simulink model "DCV_test"  (R2025b)
settings: Solver=VariableStepAuto  StartTime=0.0  StopTime=10.0  RelTol=1e-3
model workspace (MATLAB code in the model file):
  | clear;
  | %% Hydraulics
  | 
  | %Liquid
  | rho = 875;
  | beta = 1000; %MPa
  | 
  | %Pump
  | pP = 10e6; %100 bar i pascal, velger den sjøl med å skru
  | 
  | %-------------------DCV-----------------------
  | dp0 = 20e5; %Nominal pressure drop, Pa
  | Q0 = 18/6e4; %Nominal flow, m^3/s
  | Cd = 0.55; %Discharge coefficient
  | AdMax_SI = Q0/(Cd*(2/rho*dp0)^0.5); %Discharge area m^2
  | AdMax = AdMax_SI*1e6;
  | 
  | %% DCV Orifice Area Vectors
  | 
  | % Deadband control signal thresholds
  | u_dead_up    = 0.236;
  | u_dead_down  = 0.206;
  | 
  | % Spool position at deadband
  | spool_dead_up   = 1.1182 * u_dead_up   - 0.0325;
  | spool_dead_down = 1.1075 * u_dead_down - 0.0416;
  | 
  | % Polynomial: spool position as function of Kv [L/min/sqrt(bar)]
  | % Valid from u = 0.25 to max stroke
  | p_spool_of_Kv_up   = [0.0018653, -0.033672,  0.22033, -0.65618,  0.83411, -0.047269, 0.26252];
  | p_spool_of_Kv_down = [0.00098272, -0.017507,  0.11599, -0.34851,  0.41222,  0.17643,  0.2076];
  | 
  | % Linear model slopes (from TwinCAT): spool_pos = spool_dead + slope * Kv
  | slope_Kv_up   = 0.270407;
  | slope_Kv_down = 0.230397;
  | 
  | % Evaluate polynomial over valid Kv range
  | Kv_range   = linspace(0.09, 4, 10000);
  | spool_up   = polyval(p_spool_of_Kv_up,   Kv_range);
  | spool_down = polyval(p_spool_of_Kv_down, Kv_range);
  | 
  | % Breakpoints: u = 0.25 to 0.50 in steps of 0.05, then max
  | %u_breakpoints = 0.25:0.05:1.0; tester flere punkter
  | u_breakpoints = [0.25, 0.30:0.025:1.0];
  | 
  | % Corresponding spool positions
  | spool_bp_up   = 1.1182 * u_breakpoints - 0.0325;
  | spool_bp_down = 1.1075 * u_breakpoints - 0.0416;
  | 
  | % Find Kv at each breakpoint using nearest-index lookup
  | Kv_bp_up   = zeros(1, length(u_breakpoints));
  | Kv_bp_down = zeros(1, length(u_breakpoints));
  | for i = 1:length(u_breakpoints)
  |     if u_breakpoints(i) <= 0.25
  |         % Use linear model for transition point
  |         Kv_bp_up(i)   = (spool_bp_up(i)   - spool_dead_up)   / slope_Kv_up;
  |         Kv_bp_down(i) = (spool_bp_down(i) - spool_dead_down) / slope_Kv_down;
  |     else
  |         % Use polynomial inversion via nearest-index lookup
  |         [~, idx_up]   = min(abs(spool_up   - spool_bp_up(i)));
  |         [~, idx_down] = min(abs(spool_down - spool_bp_down(i)));
  |         Kv_bp_up(i)   = Kv_range(idx_up);
  |         Kv_bp_down(i) = Kv_range(idx_down);
  |     end
  | end
  | 
  | % Kv at max spool
  | [~, idx_max_up]   = max(spool_up);
  | [~, idx_max_down] = max(spool_down);
  | Kv_max_up   = Kv_range(idx_max_up);
  | Kv_max_down = Kv_range(idx_max_down);
  | 
  | % Unit conversion: L/min/sqrt(bar) -> m³/s/sqrt(Pa)
  | Kv_unit_conv = sqrt(1e-5) / 6e4;
  | 
  | % Convert all Kv breakpoints to area [m²]
  | A_bp_up   = (Kv_bp_up   * Kv_unit_conv) / (Cd * sqrt(2/rho));
  | A_bp_down = (Kv_bp_down * Kv_unit_conv) / (Cd * sqrt(2/rho));
  | A_max_up  = (Kv_max_up  * Kv_unit_conv) / (Cd * sqrt(2/rho));
  | A_max_down= (Kv_max_down* Kv_unit_conv) / (Cd * sqrt(2/rho));
  | 
  | % Orifice area vectors [m²]: [leakage, crack-open, u=0.30...0.50, fully-open]
  | orifice_area_up   = [1e-9, A_bp_up,   A_max_up];
  | orifice_area_down = [1e-9, A_bp_down, A_max_down];
  | 
  | % Control member position vectors (must match area vectors one-to-one)
  | u_max_pos = 1.05; % position for max area point, beyond valid range to avoid duplicate
  | % control_pos_up   = [0, u_breakpoints, u_max_pos]; gamle måtte fikse
  | % control_pos_down = [0, u_breakpoints, u_max_pos];
  | 
  | control_pos_up   = [0, spool_bp_up,   1.1182 * u_max_pos - 0.0325];
  | control_pos_down = [0, spool_bp_down, 1.1075 * u_max_pos - 0.0416];
  | 
  | % ------------------CBV-------------------
  | alpha = 5; %Pilot ratio
  | pCr_A = 245; %Bar, har tatt verdier fra rød kran, Dette må måles da vi ikek vet.
  | dp_open_A = 245; %Bar setter lik pcrack først
  | 
  | Cd_CBV = 0.8;
  | AdMax_CBV = (60 / 6e4) / sqrt(2/rho * 16e5) / Cd_CBV; %SJekk over denne
  | 
  | %% Test orifice
  | u_test = 0.8;
  | 
  | spool_test_up   = 1.1182 * u_test - 0.0325;
  | spool_test_down = 1.1075 * u_test - 0.0416;
  | 
  | [~, idx_up]   = min(abs(spool_up   - spool_test_up));
  | [~, idx_down] = min(abs(spool_down - spool_test_down));
  | 
  | Kv_expected_up   = Kv_range(idx_up);
  | Kv_expected_down = Kv_range(idx_down);
libraries: fl_lib x6, nesl_utility x4, SimscapeFluids_lib x2
settings Model: Creator=sujro  LastModifiedBy=sujro

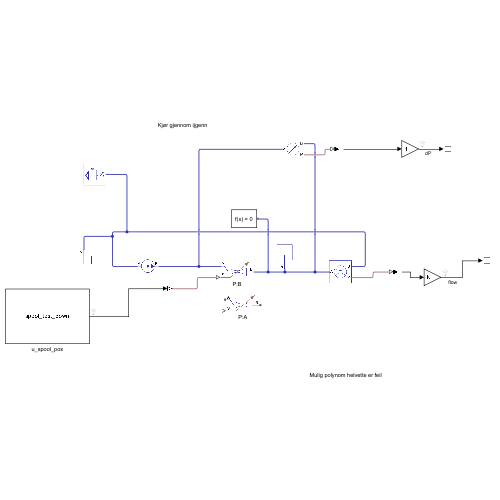
[thumbnail: Simulink's stored preview of the top-level diagram]
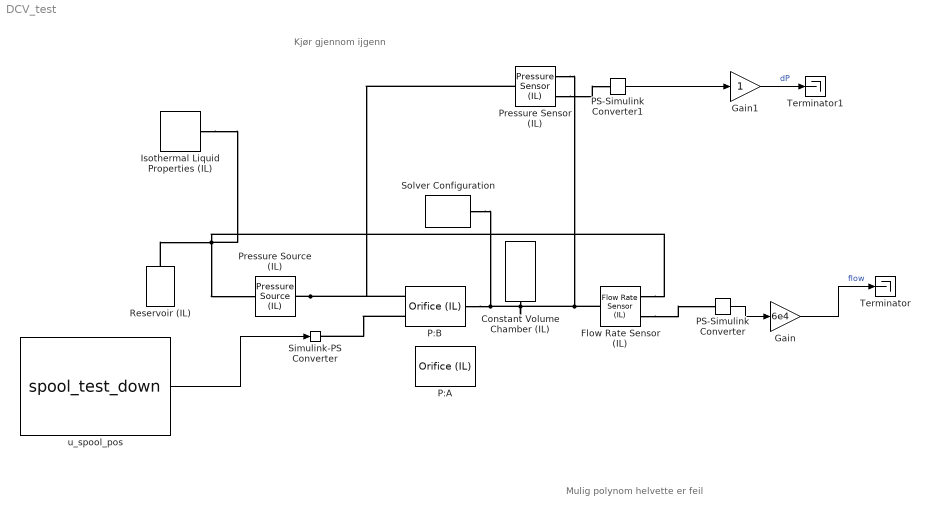
== system DCV_test ==
  note: Kjør gjennom ijgenn
  note: Mulig polynom helvette er feil
  Constant Volume Chamber (IL) : fl_lib/Isothermal Liquid/Elements/Constant Volume Chamber (IL)  volume=0.001 m^3  p_I_specify=off  p_I_priority=High  p_I=0.101325 MPa  p_I_nominal_specify=off  p_I_nominal_value=1  p_I_nominal_unit=MPa
      settings: InternalSimscapePortConfiguration="{\"Bottom\":[],\"Left\":[{\"id\":\"A\",\"label\":\"A\",\"type\":\"foundation.isothermal_liquid.isothermal_liquid\"}],\"Right\":[],\"Top\":[]}"
  Flow Rate Sensor (IL) : fl_lib/Isothermal Liquid/Sensors/Flow Rate Sensor (IL)  sensor_type=foundation.enum.mass_volumetric_sensor.volumetric
      settings: InternalSimscapePortConfiguration="{\"Bottom\":[],\"Left\":[{\"id\":\"A\",\"label\":\"A\",\"type\":\"foundation.isothermal_liquid.isothermal_liquid\"}],\"Right\":[{\"id\":\"B\",\"label\":\"B\",\"type\":\"foundation.isothermal_liquid.isothermal_liquid\"},{\"id\":\"V\",\"label\":\"V\",\"type\":\"output\"}],\"Top\":[]}"
  Gain : Gain  Gain=6e4
  Gain1 : Gain
  Isothermal Liquid Properties (IL) : fl_lib/Isothermal Liquid/Utilities/Isothermal Liquid Properties (IL)  rho_L_atm=rho kg/m^3  bulk_modulus_model=foundation.enum.bulk_modulus_model.const  beta_gain=6  beta_L_atm=beta MPa  nu_atm=1.0034e-6 m^2/s  p_atm=0.101325 MPa  p_min=1 Pa  properties_range_check=simscape.enum.assert.action.error  air_fraction=0.005  polytropic_index=1.0  rho_g_atm=1.225 kg/m^3  air_dissolution_model=false  p_crit=3 MPa
  P:A : SimscapeFluids_lib/Isothermal Liquid/Valves & Orifices/Orifices/Orifice (IL)  orifice_type=foundation.enum.constant_variable.variable  constant_orifice_spec=fluids.isothermal_liquid.valves_orifices.orifices.enum.constant_orifice_spec.area  variable_orifice_spec=fluids.isothermal_liquid.valves_orifices.orifices.enum.orifice_spec.table1D_area_opening  orifice_area_constant=1e-3 m^2  p_diff_TLU_constant=[-4, -3, -2, -1, -.5, 0, .5, 1, 2, 3, 4] MPa  vol_flow_TLU_constant=[-2.44, -2.12, -1.68, -1.22, -.84, 0, .85, 1.21, 1.7, 2.09, 2.41] .* 1e-3 m^3/s  S_min=0 m  del_S=1 m  open_orientation=fluids.isothermal_liquid.valves_orifices.orifices.enum.orifice_orientation.positive  area_max=A_max_up m^2  area_leak=1e-10 m^2  S_TLU=control_pos_up m  orifice_area_TLU=orifice_area_up m^2  area=inf m^2  Cd=Cd  Re_c=150  smoothing_factor=0.01  pressure_recovery=false  S_vol_flow_TLU=[0, .002, .004, .007, .017] m  p_diff_TLU=[.3, .5, .7] MPa  vol_flow_TLU=1e-3 * [1.7e-05, 2e-05, 2.6e-05; .0035, .0045, .0053; .7, .9, 1.06; 1.96, 2.5, 3; 6, 7.7, 9.13] m^3/s
      settings: InternalSimscapePortConfiguration="{\"Bottom\":[],\"Left\":[{\"id\":\"A\",\"label\":\"A\",\"type\":\"foundation.isothermal_liquid.isothermal_liquid\"},{\"id\":\"S\",\"label\":\"S\",\"type\":\"input\"}],\"Right\":[{\"id\":\"B\",\"label\":\"B\",\"type\":\"foundation.isothermal_liquid.isothermal_liquid\"}],\"Top\":[]}"
  P:B : SimscapeFluids_lib/Isothermal Liquid/Valves & Orifices/Orifices/Orifice (IL)  orifice_type=foundation.enum.constant_variable.variable  constant_orifice_spec=fluids.isothermal_liquid.valves_orifices.orifices.enum.constant_orifice_spec.area  variable_orifice_spec=fluids.isothermal_liquid.valves_orifices.orifices.enum.orifice_spec.table1D_area_opening  orifice_area_constant=1e-3 m^2  p_diff_TLU_constant=[-4, -3, -2, -1, -.5, 0, .5, 1, 2, 3, 4] MPa  vol_flow_TLU_constant=[-2.44, -2.12, -1.68, -1.22, -.84, 0, .85, 1.21, 1.7, 2.09, 2.41] .* 1e-3 m^3/s  S_min=0 m  del_S=1 m  open_orientation=fluids.isothermal_liquid.valves_orifices.orifices.enum.orifice_orientation.positive  area_max=A_max_down m^2  area_leak=1e-10 m^2  S_TLU=control_pos_down m  orifice_area_TLU=orifice_area_down m^2  area=inf m^2  Cd=Cd  Re_c=0.01  smoothing_factor=0.01  pressure_recovery=false  S_vol_flow_TLU=[0, .002, .004, .007, .017] m  p_diff_TLU=[.3, .5, .7] MPa  vol_flow_TLU=1e-3 * [1.7e-05, 2e-05, 2.6e-05; .0035, .0045, .0053; .7, .9, 1.06; 1.96, 2.5, 3; 6, 7.7, 9.13] m^3/s
      settings: InternalSimscapePortConfiguration="{\"Bottom\":[],\"Left\":[{\"id\":\"A\",\"label\":\"A\",\"type\":\"foundation.isothermal_liquid.isothermal_liquid\"},{\"id\":\"S\",\"label\":\"S\",\"type\":\"input\"}],\"Right\":[{\"id\":\"B\",\"label\":\"B\",\"type\":\"foundation.isothermal_liquid.isothermal_liquid\"}],\"Top\":[]}"
  PS-Simulink Converter : nesl_utility/PS-Simulink Converter  PhysicalDomain=network_engine_domain  SubClassName=ps_output  LeftPortType=input  RightPortType=output  PseudoPeriodic=off  Frequencies=[]  VectorFormat=inherit  Unit=inherit  AffineConversion=off
  PS-Simulink Converter1 : nesl_utility/PS-Simulink Converter  PhysicalDomain=network_engine_domain  SubClassName=ps_output  LeftPortType=input  RightPortType=output  PseudoPeriodic=off  Frequencies=[]  VectorFormat=inherit  Unit=inherit  AffineConversion=off
  Pressure Sensor (IL) : fl_lib/Isothermal Liquid/Sensors/Pressure Sensor (IL)  pressure_measure=foundation.enum.pressure_measure.difference
      settings: InternalSimscapePortConfiguration="{\"Bottom\":[],\"Left\":[{\"id\":\"A\",\"label\":\"A\",\"type\":\"foundation.isothermal_liquid.isothermal_liquid\"}],\"Right\":[{\"id\":\"B\",\"label\":\"B\",\"type\":\"foundation.isothermal_liquid.isothermal_liquid\"},{\"id\":\"P\",\"label\":\"P\",\"type\":\"output\"}],\"Top\":[]}"
  Pressure Source (IL) : fl_lib/Isothermal Liquid/Sources/Pressure Source (IL)  source_type=foundation.enum.constant_controlled.constant  pressure_differential=1 bar
      settings: InternalSimscapePortConfiguration="{\"Bottom\":[],\"Left\":[{\"id\":\"A\",\"label\":\"A\",\"type\":\"foundation.isothermal_liquid.isothermal_liquid\"}],\"Right\":[{\"id\":\"B\",\"label\":\"B\",\"type\":\"foundation.isothermal_liquid.isothermal_liquid\"}],\"Top\":[]}"
  Reservoir (IL) : fl_lib/Isothermal Liquid/Elements/Reservoir (IL)  reservoir_type=foundation.enum.constant_controlled.constant  pressure_spec=foundation.enum.pressure_spec.atmospheric  reservoir_pressure=0 MPa
  Simulink-PS Converter : nesl_utility/Simulink-PS Converter  PhysicalDomain=network_engine_domain  SubClassName=ps_input  LeftPortType=input  RightPortType=output  PseudoPeriodic=off  Frequencies=[]  NoiseDistribution=none  NoiseParameters=[]  Unit=1  AffineConversion=off  FilteringAndDerivatives=provide  SimscapeFilterOrder=1  InputFilterTimeConstant=0.001  UdotUserProvided=0
  Solver Configuration : nesl_utility/Solver Configuration  PhysicalDomain=network_engine_domain  SubClassName=solver  LeftPortType=input  RightPortType=generic  Tones=[]  Harmonics=[]  SimulateNoise=off  Profile=off  UseLocalSampling=off  EnableSwitchedLinearOptims=on  FrequencyDomain=off  UseCCode=off  RelTol=0.001  AbsTol=0.001  MinStep=1e-09  ToWorkspace=off  RevertToSquareIcSolve=off  NumHomotopyIterations=100  PhasorMode=off  PhasorModeNumHarmonics=1  ConsistencySolver=NEWTON_XTOL_AFTER_FTOL  IndexReductionMethod=DerivativeReplacement  DoDC=off  ResidualTolerance=1e-09  ConsistencyTolSource=GLOBAL  ConsistencyAbsTol=0.001  ConsistencyRelTol=0.001  ConsistencyTolFactor=0.001  UseLocalSolver=off  LocalSolverChoice=NE_BACKWARD_EULER_ADVANCER  ResolveIndetEquations=on  FunctionEvalNumThread=1  LocalSolverSampleTime=0.001  DoFixedCost=off  MaxNonlinIter=3  MaxModeIter=2  ComputeImpulses=off  ImpulseIterations=2  LinearAlgebra=auto  LinearAlgebraNumThread=0  EquationFormulation=NE_TIME_EF  DelaysMemoryBudget=1024  AutomaticFiltering=on  FilteringTimeConstant=0.001  PartitionStorageMethod=AS_NEEDED  PartitionMemoryBudget=1024  PartitionMethod=ROBUST  MultibodyUseLocalSolver=off  MultibodyLocalSolverChoice=ODE1  MultibodyLocalSolverSampleTime=0.001
  Terminator : Terminator
  Terminator1 : Terminator
  u_spool_pos : Constant  Value=spool_test_down
  wires:
  Gain/1 -> Terminator/1  "flow"
  PS-Simulink Converter/1 -> Gain/1
  u_spool_pos/1 -> Simulink-PS Converter/1
  PS-Simulink Converter1/1 -> Gain1/1
  Gain1/1 -> Terminator1/1  "dP"
  connections:
  Flow Rate Sensor (IL)/LConn1 -- Constant Volume Chamber (IL)/LConn1 -- P:B/RConn1 -- Solver Configuration/RConn1 -- Pressure Sensor (IL)/RConn1
  Pressure Source (IL)/RConn1 -- P:B/LConn1 -- Pressure Sensor (IL)/LConn1
  P:B/LConn2 -- Simulink-PS Converter/RConn1
  Reservoir (IL)/LConn1 -- Isothermal Liquid Properties (IL)/RConn1 -- Flow Rate Sensor (IL)/RConn1 -- Pressure Source (IL)/LConn1
  Flow Rate Sensor (IL)/RConn2 -- PS-Simulink Converter/LConn1
  Pressure Sensor (IL)/RConn2 -- PS-Simulink Converter1/LConn1
